simulink model "measurementTesting"  (R2025a)
settings: Solver=VariableStepAuto  StartTime=0.0  StopTime=30  RelTol=1e-3
model workspace (MATLAB code in the model file):
  | Ts = 0.0001
undefined symbols (not defined in the file or in its folder): canChannel, SampleTime
libraries: canlib x4, eeGeneralControl x4, canmsglib x3, simulink x1
settings Model: Creator=eliasalbag  LastModifiedBy=eliasalbag

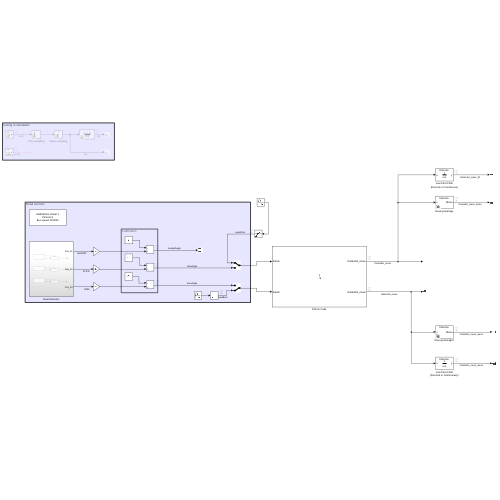
[thumbnail: Simulink's stored preview of the top-level diagram]
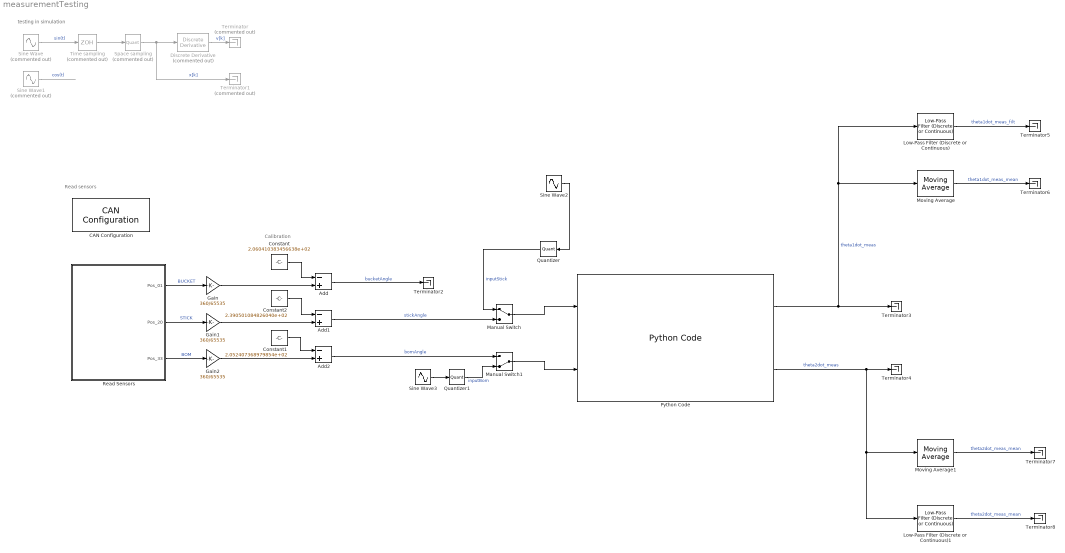
== system measurementTesting ==
  note: testing in simulation
  note: Calibration
  note: Read sensors
  Add : Sum  Inputs=-+
  Add1 : Sum  Inputs=-+
  Add2 : Sum  Inputs=-+
  CAN Configuration : canlib/CAN Configuration  BlockHandle=1689.0001  Device=MathWorks Virtual 1 (Channel 1)  DeviceMenu=MathWorks Virtual 1 (Channel 1)  ObjConstructor=canChannel('MathWorks', 'Virtual 1', 1)  BusSpeed=500000  EnableBitParameters=off  AckMode=Normal
  Constant : Constant  Value=2.060410383456638e+02
  Constant1 : Constant  Value=2.052407368979854e+02
  Constant2 : Constant  Value=2.390501084826040e+02
  Discrete Derivative : simulink/Discrete/Discrete Derivative  Commented=on  gainval=1.0  ICPrevScaledInput=0.0  OutMin=[]  OutMax=[]  OutDataType=fixdt(1, 16)  OutScaling=2^-10  DoSatur=off
  Gain : Gain  Gain=360/65535
  Gain1 : Gain  Gain=360/65535
  Gain2 : Gain  Gain=360/65535
  Low-Pass Filter (Discrete or Continuous) : eeGeneralControl/Low-Pass Filter (Discrete or Continuous)  K=1  T=1  B=inf  A=-inf  init_option=Specify as parameter  x0=0  Ts=Ts
  Low-Pass Filter (Discrete or Continuous)1 : eeGeneralControl/Low-Pass Filter (Discrete or Continuous)  K=1  T=1  B=inf  A=-inf  init_option=Specify as parameter  x0=0  Ts=Ts
  Manual Switch : ManualSwitch
  Manual Switch1 : ManualSwitch  CurrentSetting=0
  Moving Average : eeGeneralControl/Moving Average  VariantControl=Variant1  LabelModeActiveChoice=Discrete  f=60  x0=0  BufferSize=8192  Ts=Ts
      settings: LibrarySourceBlock=ee_sl_lib/General Control/Moving Average
  Moving Average1 : eeGeneralControl/Moving Average  VariantControl=Variant1  LabelModeActiveChoice=Discrete  f=60  x0=0  BufferSize=8192  Ts=Ts
      settings: LibrarySourceBlock=ee_sl_lib/General Control/Moving Average
  Python Code : PythonCode  OutputCode=|  SampleTime=SampleTime  DT=Ts  SampleTime=Ts
      | #code for testing how the numerical derivation is affected by sampling time etc.
      | #change sampling time to see how the derivated output is affected
      | 
      | 
      | if theta1_prev is None:
      |     theta1_prev = 0.0
      | if theta2_prev is None:
      |     theta2_prev = 0.0
      | 
      | #raw derivative calculation
      | #DT is a parameter
      | theta1dot_meas = (theta1 - theta1_prev) / DT
      | theta2dot_meas = (theta2 - theta2_prev) / DT
      | 
      | theta1_prev = theta1
      | theta2_prev = theta2
  Quantizer : Quantizer  QuantizationInterval=2*pi/(2^16-1)
  Quantizer1 : Quantizer  QuantizationInterval=2*pi/(2^16-1)
  Read Sensors : Subsystem
  Sine Wave : Sin  Commented=on  SampleTime=0
  Sine Wave1 : Sin  Commented=on  Phase=pi/2  SampleTime=0
  Sine Wave2 : Sin  SampleTime=0
  Sine Wave3 : Sin  Phase=pi/2  SampleTime=0
  Space sampling : Quantizer  Commented=on  QuantizationInterval=2*pi/(2^15-1)
  Terminator : Terminator  Commented=on
  Terminator1 : Terminator  Commented=on
  Terminator{2..8} (7 alike) : Terminator
  Time sampling : ZeroOrderHold  Commented=on  SampleTime=1e-2
  wires:
  Sine Wave1/1 -> ?  "cos(t)"
  Sine Wave/1 -> Time sampling/1  "sin(t)"
  Space sampling/1 -> Terminator1/1, Discrete Derivative/1  "x[k]"
  Time sampling/1 -> Space sampling/1
  Discrete Derivative/1 -> Terminator/1  "v[k]"
  Read Sensors/1(Pos_01) -> Gain/1  "BUCKET"
  Read Sensors/2(Pos_20) -> Gain1/1  "STICK"
  Gain2/1 -> Add2/2
  Read Sensors/3(Pos_33) -> Gain2/1  "BOM"
  Add2/1 -> Manual Switch1/1  "bomAngle"
  Constant1/1 -> Add2/1
  Gain1/1 -> Add1/2
  Gain/1 -> Add/2
  Add/1 -> Terminator2/1  "bucketAngle"
  Add1/1 -> Manual Switch/2  "stickAngle"
  Constant/1 -> Add/1
  Constant2/1 -> Add1/1
  Python Code/1 -> Low-Pass Filter (Discrete or Continuous)/1, Moving Average/1, Terminator3/1  "theta1dot_meas"
  Python Code/2 -> Low-Pass Filter (Discrete or Continuous)1/1, Moving Average1/1, Terminator4/1  "theta2dot_meas"
  Sine Wave2/1 -> Quantizer/1
  Manual Switch/1 -> Python Code/1
  Manual Switch1/1 -> Python Code/2
  Sine Wave3/1 -> Quantizer1/1
  Low-Pass Filter (Discrete or Continuous)/1 -> Terminator5/1  "theta1dot_meas_filt"
  Moving Average/1 -> Terminator6/1  "theta1dot_meas_mean"
  Moving Average1/1 -> Terminator7/1  "theta2dot_meas_mean"
  Low-Pass Filter (Discrete or Continuous)1/1 -> Terminator8/1  "theta2dot_meas_mean"
  Quantizer/1 -> Manual Switch/1  "inputStick"
  Quantizer1/1 -> Manual Switch1/2  "inputBom"

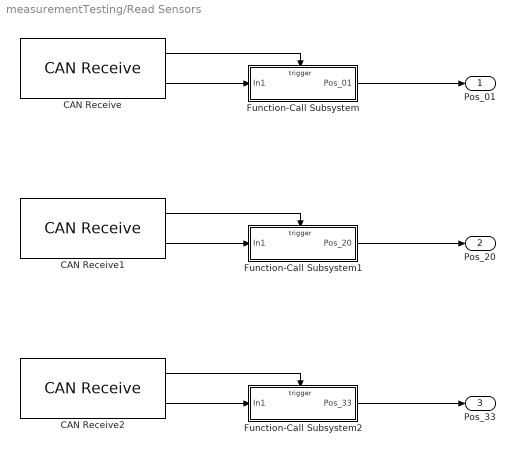
== system measurementTesting/Read Sensors ==
  CAN Receive : canlib/CAN Receive  BlockHandle=2343.0002  Device=MathWorks Virtual 1 (Channel 1)  DeviceMenu=MathWorks Virtual 1 (Channel 1)  ObjConstructor=canChannel('MathWorks', 'Virtual 1', 1)  EnableStandardIDsFilter=off  StdIDsCombo=Allow all  StandardIDs=0  EnableExtendedIDsFilter=off  ExtIDsCombo=Allow all  ExtendedIDs=0  SampleTime=0.01  MsgsPerTimestep=all  InternalFilterUpdateStatus=on  BusOutput=off
  CAN Receive1 : canlib/CAN Receive  BlockHandle=2346.0001  Device=MathWorks Virtual 1 (Channel 1)  DeviceMenu=MathWorks Virtual 1 (Channel 1)  ObjConstructor=canChannel('MathWorks', 'Virtual 1', 1)  EnableStandardIDsFilter=off  StdIDsCombo=Allow all  StandardIDs=0  EnableExtendedIDsFilter=off  ExtIDsCombo=Allow all  ExtendedIDs=0  SampleTime=0.01  MsgsPerTimestep=all  InternalFilterUpdateStatus=on  BusOutput=off
  CAN Receive2 : canlib/CAN Receive  BlockHandle=2349.0001  Device=MathWorks Virtual 1 (Channel 1)  DeviceMenu=MathWorks Virtual 1 (Channel 1)  ObjConstructor=canChannel('MathWorks', 'Virtual 1', 1)  EnableStandardIDsFilter=off  StdIDsCombo=Allow all  StandardIDs=0  EnableExtendedIDsFilter=off  ExtIDsCombo=Allow all  ExtendedIDs=0  SampleTime=0.01  MsgsPerTimestep=all  InternalFilterUpdateStatus=on  BusOutput=off
  Function-Call Subsystem : Subsystem  TreatAsAtomicUnit=on
  Function-Call Subsystem1 : Subsystem  TreatAsAtomicUnit=on
  Function-Call Subsystem2 : Subsystem  TreatAsAtomicUnit=on
  Pos_01 : Outport
  Pos_20 : Outport  Port=2
  Pos_33 : Outport  Port=3
  wires:
  CAN Receive/2 -> Function-Call Subsystem/1(In1)
  CAN Receive1/2 -> Function-Call Subsystem1/1(In1)
  CAN Receive/1 -> Function-Call Subsystem/Trigger
  CAN Receive2/2 -> Function-Call Subsystem2/1(In1)
  Function-Call Subsystem2/1(Pos_33) -> Pos_33/1
  Function-Call Subsystem/1(Pos_01) -> Pos_01/1
  CAN Receive2/1 -> Function-Call Subsystem2/Trigger
  CAN Receive1/1 -> Function-Call Subsystem1/Trigger
  Function-Call Subsystem1/1(Pos_20) -> Pos_20/1

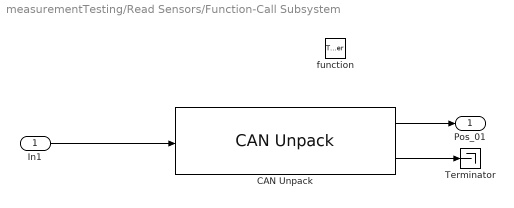
== system measurementTesting/Read Sensors/Function-Call Subsystem ==
  In1 : Inport
  function : TriggerPort  TriggerType=function-call  VariantControl=(inherit)
  CAN Unpack : canmsglib/CAN Unpack  CANdbFile=C:\Users\Viktor Traktor\Downloads\VolvoExcavator\systemIdentificationVolvo\ec20_kth.dbc  MsgList=Rot_01  MsgName=Rot_01  MsgIDType=Extended (29-bit identifier)  MsgIdentifier=419408385  MsgLength=8  SignalInfo={'SnsrPos_01','0','32','LE','unsigned','Standard','0','1','0','0','4294967295';'SnsrRPM_01','32','16','LE','unsigned','Standard','0','1','0','0','65535'}  IDPort=off  TimestampPort=off  ErrorPort=off  RemotePort=off  LengthPort=off  StatusPort=off  ApplyMinMax=off
      settings: LibrarySourceBlock=canlib/CAN Unpack  DataFormat=CANdb specified signals
  Terminator : Terminator
  Pos_01 : Outport
  wires:
  In1/1 -> CAN Unpack/1
  CAN Unpack/1 -> Pos_01/1
  CAN Unpack/2 -> Terminator/1

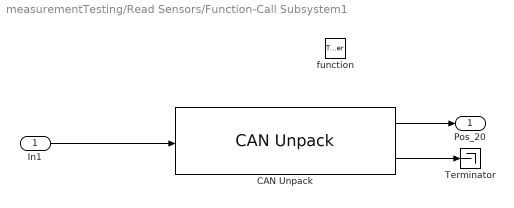
== system measurementTesting/Read Sensors/Function-Call Subsystem1 ==
  In1 : Inport
  function : TriggerPort  TriggerType=function-call  VariantControl=(inherit)
  CAN Unpack : canmsglib/CAN Unpack  CANdbFile=C:\Users\Viktor Traktor\Downloads\VolvoExcavator\systemIdentificationVolvo\ec20_kth.dbc  MsgList=Rot_20  MsgName=Rot_20  MsgIDType=Extended (29-bit identifier)  MsgIdentifier=419408416  MsgLength=8  SignalInfo={'SnsrPos_20','0','32','LE','unsigned','Standard','0','1','0','0','4294967295';'SnsrRPM_20','32','16','LE','unsigned','Standard','0','1','0','0','65535'}  IDPort=off  TimestampPort=off  ErrorPort=off  RemotePort=off  LengthPort=off  StatusPort=off  ApplyMinMax=off
      settings: LibrarySourceBlock=canlib/CAN Unpack  DataFormat=CANdb specified signals
  Terminator : Terminator
  Pos_20 : Outport
  wires:
  CAN Unpack/1 -> Pos_20/1
  In1/1 -> CAN Unpack/1
  CAN Unpack/2 -> Terminator/1

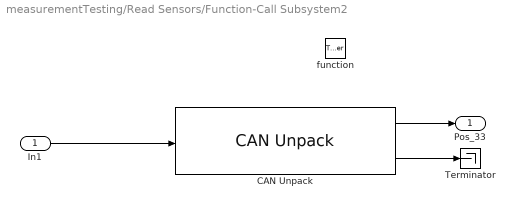
== system measurementTesting/Read Sensors/Function-Call Subsystem2 ==
  In1 : Inport
  function : TriggerPort  TriggerType=function-call  VariantControl=(inherit)
  CAN Unpack : canmsglib/CAN Unpack  CANdbFile=C:\Users\Viktor Traktor\Downloads\VolvoExcavator\systemIdentificationVolvo\ec20_kth.dbc  MsgList=Rot_33  MsgName=Rot_33  MsgIDType=Extended (29-bit identifier)  MsgIdentifier=419408435  MsgLength=8  SignalInfo={'SnsrPos_33','0','32','LE','unsigned','Standard','0','1','0','0','4294967295';'SnsrRPM_33','32','16','LE','unsigned','Standard','0','1','0','0','65535'}  IDPort=off  TimestampPort=off  ErrorPort=off  RemotePort=off  LengthPort=off  StatusPort=off  ApplyMinMax=off
      settings: LibrarySourceBlock=canlib/CAN Unpack  DataFormat=CANdb specified signals
  Terminator : Terminator
  Pos_33 : Outport
  wires:
  In1/1 -> CAN Unpack/1
  CAN Unpack/1 -> Pos_33/1
  CAN Unpack/2 -> Terminator/1
